simulink model "MasaResorte"  (R2021b)
settings: Solver=VariableStepAuto  StartTime=0.0  StopTime=2  RelTol=1e-3
settings Model: Creator=juandiegocastropadilla  LastModifiedBy=juandiegocastropadilla

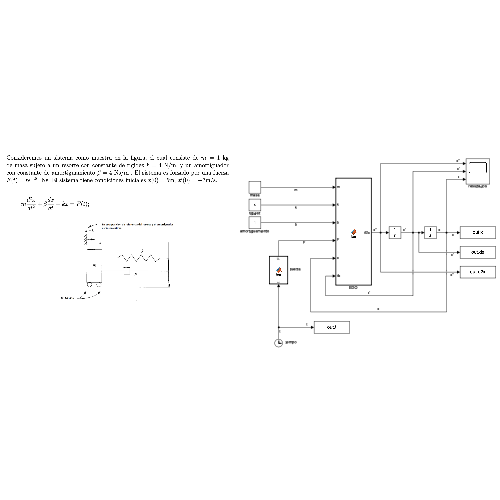
[thumbnail: Simulink's stored preview of the top-level diagram]
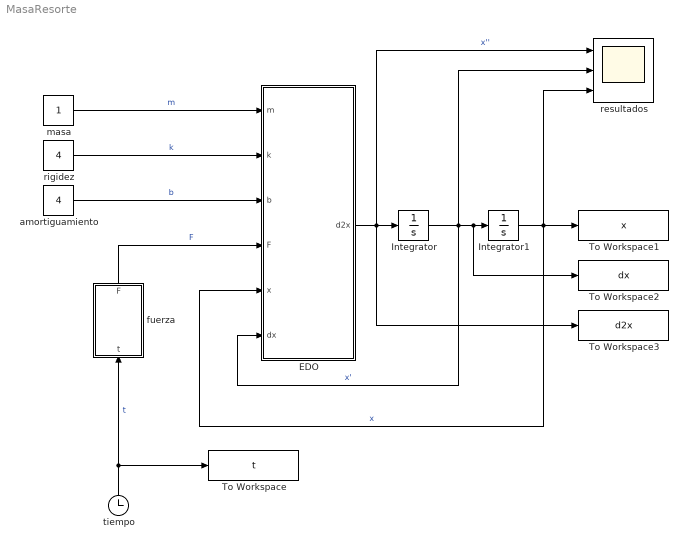
== system MasaResorte ==
  EDO : MATLAB Function  TreatAsAtomicUnit=on
  Integrator : Integrator  InitialCondition=-7
  Integrator1 : Integrator  InitialCondition=5
  To Workspace : ToWorkspace  VariableName=t  SampleTime=-1
  To Workspace1 : ToWorkspace  VariableName=x  SampleTime=-1
  To Workspace2 : ToWorkspace  VariableName=dx  SampleTime=-1
  To Workspace3 : ToWorkspace  VariableName=d2x  SampleTime=-1
  amortiguamiento : Constant  Value=4
  fuerza : MATLAB Function  TreatAsAtomicUnit=on
  masa : Constant
  resultados : Scope  NumInputPorts=3
  rigidez : Constant  Value=4
  tiempo : Clock
  wires:
  tiempo/1 -> To Workspace/1, fuerza/1(t)  "t"
  fuerza/1(F) -> EDO/4(F)  "F"
  masa/1 -> EDO/1(m)  "m"
  rigidez/1 -> EDO/2(k)  "k"
  amortiguamiento/1 -> EDO/3(b)  "b"
  EDO/1(d2x) -> To Workspace3/1, resultados/1, Integrator/1  "x''"
  Integrator/1 -> To Workspace2/1, Integrator1/1, EDO/6(dx), resultados/2  "x'"
  Integrator1/1 -> resultados/3, To Workspace1/1, EDO/5(x)  "x"

== matlab function MasaResorte/EDO ==
  data: m input; d2x output; k input; b input; F input; x input; dx input
function d2x = fcn(m, k, b, F, x, dx)

d2x = (F-k*x-b*dx)/m;

== matlab function MasaResorte/fuerza ==
  data: t input; F output
function F = fcn(t)

F = t.*exp(-2.*t);
